simulink model "sm_boom_lift_crawler_valve_sequence_test"  (R2026a)
settings: Solver=ode3  StopTime=46  FixedStep=2e-3
StartFcn:
  | set_param([bdroot '/Scope/Scope'],'Title',['Valve Sequence: ' tVec.SeqName]);
undefined symbols (not defined in the file or in its folder): oVec, tVec
Description:
  | Boom Lift Crawler Valve Sequence Timing
  | 
  | Copyright 2020-2026 The MathWorks(TM), Inc.
settings Model: Creator=smiller  LastModifiedBy=smiller

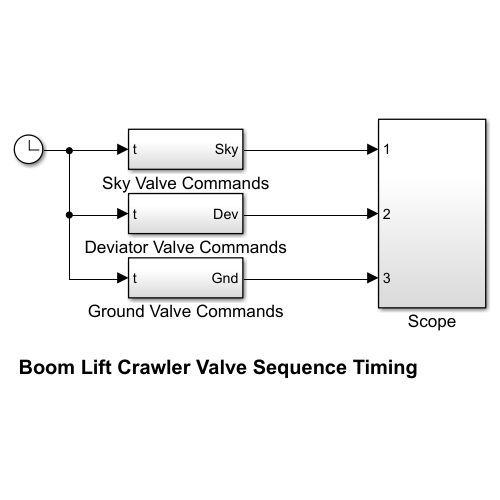
[thumbnail: Simulink's stored preview of the top-level diagram]
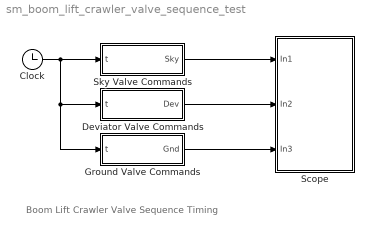
== system sm_boom_lift_crawler_valve_sequence_test ==
  note: Boom Lift Crawler Valve Sequence Timing
  Clock : Clock
  Deviator Valve Commands : Subsystem
  Ground Valve Commands : Subsystem
  Scope : Subsystem
  Sky Valve Commands : Subsystem
  wires:
  Clock/1 -> Sky Valve Commands/1(t), Deviator Valve Commands/1(t), Ground Valve Commands/1(t)
  Sky Valve Commands/1(Sky) -> Scope/1(In1)
  Deviator Valve Commands/1(Dev) -> Scope/2(In2)
  Ground Valve Commands/1(Gnd) -> Scope/3(In3)

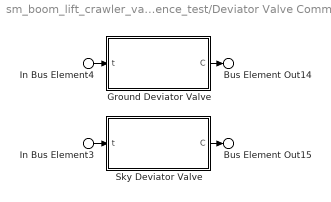
== system sm_boom_lift_crawler_valve_sequence_test/Deviator Valve Commands ==
  In Bus Element3 : Inport  PortName=t
  In Bus Element4 : Inport  PortName=t
  Ground Deviator Valve : Subsystem
  Sky Deviator Valve : Subsystem
  Bus Element Out14 : Outport  VectorParamsAs1DForOutWhenUnconnected=off  PortName=Dev  Element=g
  Bus Element Out15 : Outport  VectorParamsAs1DForOutWhenUnconnected=off  PortName=Dev  Element=s
  wires:
  In Bus Element4/1 -> Ground Deviator Valve/1(t)
  Ground Deviator Valve/1(C) -> Bus Element Out14/1
  In Bus Element3/1 -> Sky Deviator Valve/1(t)
  Sky Deviator Valve/1(C) -> Bus Element Out15/1

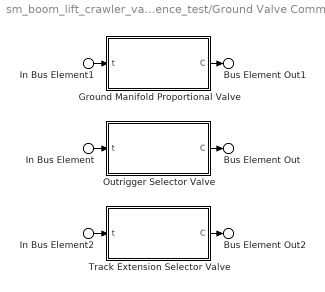
== system sm_boom_lift_crawler_valve_sequence_test/Ground Valve Commands ==
  In Bus Element : Inport  PortName=t
  In Bus Element1 : Inport  PortName=t
  In Bus Element2 : Inport  PortName=t
  Ground Manifold Proportional Valve : Subsystem
  Outrigger Selector Valve : Subsystem
  Track Extension Selector Valve : Subsystem
  Bus Element Out1 : Outport  VectorParamsAs1DForOutWhenUnconnected=off  PortName=Gnd  Element=Pr
  Bus Element Out : Outport  VectorParamsAs1DForOutWhenUnconnected=off  PortName=Gnd  Element=Ou
  Bus Element Out2 : Outport  VectorParamsAs1DForOutWhenUnconnected=off  PortName=Gnd  Element=Tr
  wires:
  In Bus Element/1 -> Outrigger Selector Valve/1(t)
  Track Extension Selector Valve/1(C) -> Bus Element Out2/1
  Ground Manifold Proportional Valve/1(C) -> Bus Element Out1/1
  In Bus Element2/1 -> Track Extension Selector Valve/1(t)
  In Bus Element1/1 -> Ground Manifold Proportional Valve/1(t)
  Outrigger Selector Valve/1(C) -> Bus Element Out/1

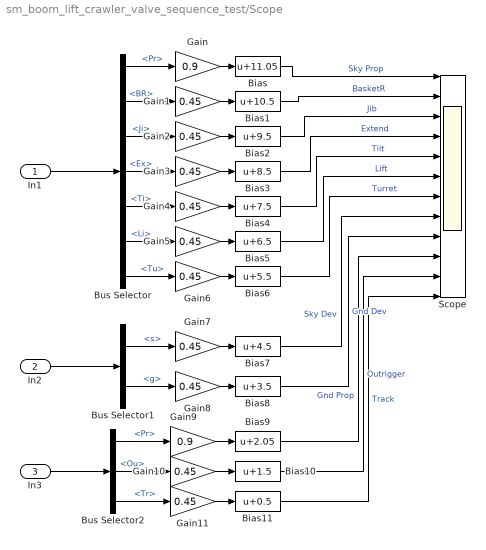
== system sm_boom_lift_crawler_valve_sequence_test/Scope ==
  In1 : Inport
  In2 : Inport  Port=2
  In3 : Inport  Port=3
  Bias : Bias  Bias=11.05  SaturateOnIntegerOverflow=off
  Bias1 : Bias  Bias=10.5  SaturateOnIntegerOverflow=off
  Bias10 : Bias  Bias=1.5  SaturateOnIntegerOverflow=off
  Bias11 : Bias  Bias=0.5  SaturateOnIntegerOverflow=off
  Bias2 : Bias  Bias=9.5  SaturateOnIntegerOverflow=off
  Bias3 : Bias  Bias=8.5  SaturateOnIntegerOverflow=off
  Bias4 : Bias  Bias=7.5  SaturateOnIntegerOverflow=off
  Bias5 : Bias  Bias=6.5  SaturateOnIntegerOverflow=off
  Bias6 : Bias  Bias=5.5  SaturateOnIntegerOverflow=off
  Bias7 : Bias  Bias=4.5  SaturateOnIntegerOverflow=off
  Bias8 : Bias  Bias=3.5  SaturateOnIntegerOverflow=off
  Bias9 : Bias  Bias=2.05  SaturateOnIntegerOverflow=off
  Bus Selector : BusSelector  OutputSignals=Pr,BR,Ji,Ex,Ti,Li,Tu
  Bus Selector1 : BusSelector  OutputSignals=s,g
  Bus Selector2 : BusSelector  OutputSignals=Pr,Ou,Tr
  Gain : Gain  Gain=0.9
  Gain{1..8,10..11} (10 alike) : Gain  Gain=0.45
  Gain9 : Gain  Gain=0.9
  Scope : Scope  NumInputPorts=12
      settings: Title=Valve Sequence: Chassis Test  ShowGrid=off  ActiveDisplayYMinimum=0  ActiveDisplayYMaximum=12
  wires:
  Gain2/1 -> Bias2/1
  Gain9/1 -> Bias9/1
  In3/1 -> Bus Selector2/1
  Bus Selector2/3 -> Gain11/1  "<Tr>"
  Bus Selector1/1 -> Gain7/1  "<s>"
  Bus Selector/6 -> Gain5/1  "<Li>"
  Gain5/1 -> Bias5/1
  Bus Selector/1 -> Gain/1  "<Pr>"
  Gain3/1 -> Bias3/1
  Gain10/1 -> Bias10/1
  Bus Selector/4 -> Gain3/1  "<Ex>"
  Gain4/1 -> Bias4/1
  Bus Selector/2 -> Gain1/1  "<BR>"
  Bus Selector2/2 -> Gain10/1  "<Ou>"
  Gain8/1 -> Bias8/1
  Gain7/1 -> Bias7/1
  Gain1/1 -> Bias1/1
  Bus Selector2/1 -> Gain9/1  "<Pr>"
  Gain6/1 -> Bias6/1
  Bus Selector/7 -> Gain6/1  "<Tu>"
  Gain/1 -> Bias/1
  Bus Selector1/2 -> Gain8/1  "<g>"
  Bus Selector/5 -> Gain4/1  "<Ti>"
  Bus Selector/3 -> Gain2/1  "<Ji>"
  Gain11/1 -> Bias11/1
  In1/1 -> Bus Selector/1
  In2/1 -> Bus Selector1/1
  Bias/1 -> Scope/1  "Sky Prop"
  Bias1/1 -> Scope/2  "BasketR"
  Bias2/1 -> Scope/3  "Jib"
  Bias3/1 -> Scope/4  "Extend"
  Bias4/1 -> Scope/5  "Tilt"
  Bias5/1 -> Scope/6  "Lift"
  Bias6/1 -> Scope/7  "Turret"
  Bias7/1 -> Scope/8  "Sky Dev"
  Bias8/1 -> Scope/9  "Gnd Dev"
  Bias9/1 -> Scope/10  "Gnd Prop"
  Bias10/1 -> Scope/11  "Outrigger"
  Bias11/1 -> Scope/12  "Track"

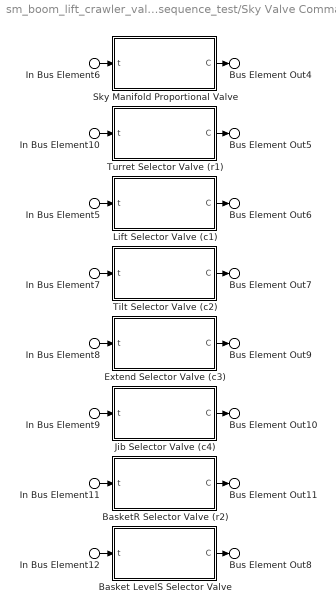
== system sm_boom_lift_crawler_valve_sequence_test/Sky Valve Commands ==
  In Bus Element{5..12} (8 alike) : Inport  PortName=t
  Basket LevelS Selector Valve : Subsystem
  BasketR Selector Valve (r2) : Subsystem
  Extend Selector Valve (c3) : Subsystem
  Jib Selector Valve (c4) : Subsystem
  Lift Selector Valve (c1) : Subsystem
  Sky Manifold Proportional Valve : Subsystem
  Tilt Selector Valve (c2) : Subsystem
  Turret Selector Valve (r1) : Subsystem
  Bus Element Out4 : Outport  VectorParamsAs1DForOutWhenUnconnected=off  PortName=Sky  Element=Pr
  Bus Element Out5 : Outport  VectorParamsAs1DForOutWhenUnconnected=off  PortName=Sky  Element=Tu
  Bus Element Out6 : Outport  VectorParamsAs1DForOutWhenUnconnected=off  PortName=Sky  Element=Li
  Bus Element Out7 : Outport  VectorParamsAs1DForOutWhenUnconnected=off  PortName=Sky  Element=Ti
  Bus Element Out8 : Outport  VectorParamsAs1DForOutWhenUnconnected=off  PortName=Sky  Element=BL
  Bus Element Out9 : Outport  VectorParamsAs1DForOutWhenUnconnected=off  PortName=Sky  Element=Ex
  Bus Element Out10 : Outport  VectorParamsAs1DForOutWhenUnconnected=off  PortName=Sky  Element=Ji
  Bus Element Out11 : Outport  VectorParamsAs1DForOutWhenUnconnected=off  PortName=Sky  Element=BR
  wires:
  In Bus Element10/1 -> Turret Selector Valve (r1)/1(t)
  BasketR Selector Valve (r2)/1(C) -> Bus Element Out11/1
  Extend Selector Valve (c3)/1(C) -> Bus Element Out9/1
  Jib Selector Valve (c4)/1(C) -> Bus Element Out10/1
  In Bus Element11/1 -> BasketR Selector Valve (r2)/1(t)
  Turret Selector Valve (r1)/1(C) -> Bus Element Out5/1
  In Bus Element12/1 -> Basket LevelS Selector Valve/1(t)
  Sky Manifold Proportional Valve/1(C) -> Bus Element Out4/1
  Basket LevelS Selector Valve/1(C) -> Bus Element Out8/1
  Lift Selector Valve (c1)/1(C) -> Bus Element Out6/1
  In Bus Element6/1 -> Sky Manifold Proportional Valve/1(t)
  In Bus Element5/1 -> Lift Selector Valve (c1)/1(t)
  In Bus Element7/1 -> Tilt Selector Valve (c2)/1(t)
  Tilt Selector Valve (c2)/1(C) -> Bus Element Out7/1
  In Bus Element9/1 -> Jib Selector Valve (c4)/1(t)
  In Bus Element8/1 -> Extend Selector Valve (c3)/1(t)

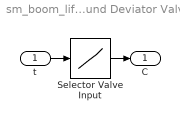
== system sm_boom_lift_crawler_valve_sequence_test/Deviator Valve Commands/Ground Deviator Valve ==
  t : Inport
  Selector Valve Input : Lookup_n-D  NumberOfTableDimensions=1  BreakpointsForDimension1=tVec.deviators.ground  Table=oVec.deviators.ground  InterpMethod=Flat  ExtrapMethod=Clip  UseLastTableValue=on  InternalRulePriority=Speed  RndMeth=Simplest
  C : Outport
  wires:
  Selector Valve Input/1 -> C/1
  t/1 -> Selector Valve Input/1

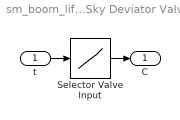
== system sm_boom_lift_crawler_valve_sequence_test/Deviator Valve Commands/Sky Deviator Valve ==
  t : Inport
  Selector Valve Input : Lookup_n-D  NumberOfTableDimensions=1  BreakpointsForDimension1=tVec.deviators.sky  Table=oVec.deviators.sky  InterpMethod=Flat  ExtrapMethod=Clip  UseLastTableValue=on  InternalRulePriority=Speed  RndMeth=Simplest
  C : Outport
  wires:
  t/1 -> Selector Valve Input/1
  Selector Valve Input/1 -> C/1

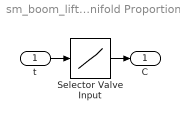
== system sm_boom_lift_crawler_valve_sequence_test/Ground Valve Commands/Ground Manifold Proportional Valve ==
  t : Inport
  Selector Valve Input : Lookup_n-D  NumberOfTableDimensions=1  BreakpointsForDimension1=tVec.ground.proportional  Table=oVec.ground.proportional  InterpMethod=Flat  ExtrapMethod=Clip  UseLastTableValue=on  InternalRulePriority=Speed  RndMeth=Simplest
  C : Outport
  wires:
  Selector Valve Input/1 -> C/1
  t/1 -> Selector Valve Input/1

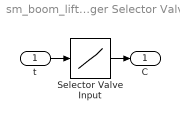
== system sm_boom_lift_crawler_valve_sequence_test/Ground Valve Commands/Outrigger Selector Valve ==
  t : Inport
  Selector Valve Input : Lookup_n-D  NumberOfTableDimensions=1  BreakpointsForDimension1=tVec.ground.c1.all  Table=oVec.ground.c1.all  InterpMethod=Flat  ExtrapMethod=Clip  UseLastTableValue=on  InternalRulePriority=Speed  RndMeth=Simplest
  C : Outport
  wires:
  t/1 -> Selector Valve Input/1
  Selector Valve Input/1 -> C/1

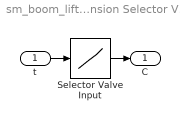
== system sm_boom_lift_crawler_valve_sequence_test/Ground Valve Commands/Track Extension Selector Valve ==
  t : Inport
  Selector Valve Input : Lookup_n-D  NumberOfTableDimensions=1  BreakpointsForDimension1=tVec.ground.c5.all  Table=oVec.ground.c5.all  InterpMethod=Flat  ExtrapMethod=Clip  UseLastTableValue=on  InternalRulePriority=Speed  RndMeth=Simplest
  C : Outport
  wires:
  Selector Valve Input/1 -> C/1
  t/1 -> Selector Valve Input/1

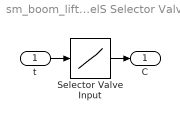
== system sm_boom_lift_crawler_valve_sequence_test/Sky Valve Commands/Basket LevelS Selector Valve ==
  t : Inport
  Selector Valve Input : Lookup_n-D  NumberOfTableDimensions=1  BreakpointsForDimension1=[0 1]  Table=[0 0]  InterpMethod=Flat  ExtrapMethod=Clip  UseLastTableValue=on  InternalRulePriority=Speed  RndMeth=Simplest
  C : Outport
  wires:
  t/1 -> Selector Valve Input/1
  Selector Valve Input/1 -> C/1

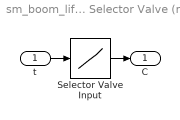
== system sm_boom_lift_crawler_valve_sequence_test/Sky Valve Commands/BasketR Selector Valve (r2) ==
  t : Inport
  Selector Valve Input : Lookup_n-D  NumberOfTableDimensions=1  BreakpointsForDimension1=tVec.sky.r2.all  Table=oVec.sky.r2.all  InterpMethod=Flat  ExtrapMethod=Clip  UseLastTableValue=on  InternalRulePriority=Speed  RndMeth=Simplest
  C : Outport
  wires:
  Selector Valve Input/1 -> C/1
  t/1 -> Selector Valve Input/1

== system sm_boom_lift_crawler_valve_sequence_test/Sky Valve Commands/Extend Selector Valve (c3) ==
  t : Inport
  Selector Valve Input : Lookup_n-D  NumberOfTableDimensions=1  BreakpointsForDimension1=tVec.sky.c3.all  Table=oVec.sky.c3.all  InterpMethod=Flat  ExtrapMethod=Clip  UseLastTableValue=on  InternalRulePriority=Speed  RndMeth=Simplest
  C : Outport
  wires:
  t/1 -> Selector Valve Input/1
  Selector Valve Input/1 -> C/1

== system sm_boom_lift_crawler_valve_sequence_test/Sky Valve Commands/Jib Selector Valve (c4) ==
  t : Inport
  Selector Valve Input : Lookup_n-D  NumberOfTableDimensions=1  BreakpointsForDimension1=tVec.sky.c4.all  Table=oVec.sky.c4.all  InterpMethod=Flat  ExtrapMethod=Clip  UseLastTableValue=on  InternalRulePriority=Speed  RndMeth=Simplest
  C : Outport
  wires:
  Selector Valve Input/1 -> C/1
  t/1 -> Selector Valve Input/1

== system sm_boom_lift_crawler_valve_sequence_test/Sky Valve Commands/Lift Selector Valve (c1) ==
  t : Inport
  Selector Valve Input : Lookup_n-D  NumberOfTableDimensions=1  BreakpointsForDimension1=tVec.sky.c1.all  Table=oVec.sky.c1.all  InterpMethod=Flat  ExtrapMethod=Clip  UseLastTableValue=on  InternalRulePriority=Speed  RndMeth=Simplest
  C : Outport
  wires:
  t/1 -> Selector Valve Input/1
  Selector Valve Input/1 -> C/1

== system sm_boom_lift_crawler_valve_sequence_test/Sky Valve Commands/Sky Manifold Proportional Valve ==
  t : Inport
  Selector Valve Input : Lookup_n-D  NumberOfTableDimensions=1  BreakpointsForDimension1=tVec.sky.proportional  Table=oVec.sky.proportional  InterpMethod=Flat  ExtrapMethod=Clip  UseLastTableValue=on  InternalRulePriority=Speed  RndMeth=Simplest
  C : Outport
  wires:
  t/1 -> Selector Valve Input/1
  Selector Valve Input/1 -> C/1

== system sm_boom_lift_crawler_valve_sequence_test/Sky Valve Commands/Tilt Selector Valve (c2) ==
  t : Inport
  Selector Valve Input : Lookup_n-D  NumberOfTableDimensions=1  BreakpointsForDimension1=tVec.sky.c2.all  Table=oVec.sky.c2.all  InterpMethod=Flat  ExtrapMethod=Clip  UseLastTableValue=on  InternalRulePriority=Speed  RndMeth=Simplest
  C : Outport
  wires:
  Selector Valve Input/1 -> C/1
  t/1 -> Selector Valve Input/1

== system sm_boom_lift_crawler_valve_sequence_test/Sky Valve Commands/Turret Selector Valve (r1) ==
  t : Inport
  Selector Valve Input : Lookup_n-D  NumberOfTableDimensions=1  BreakpointsForDimension1=tVec.sky.r1.all  Table=oVec.sky.r1.all  InterpMethod=Flat  ExtrapMethod=Clip  UseLastTableValue=on  InternalRulePriority=Speed  RndMeth=Simplest
  C : Outport
  wires:
  t/1 -> Selector Valve Input/1
  Selector Valve Input/1 -> C/1
